simulink model "block_diagram"  (R2015b)
settings: Solver=VariableStepAuto  StartTime=0.0  StopTime=10.0  RelTol=1e-3
values from neighbouring files (symbols this model uses):
  dg = [1 1]    [script.m]
  ng = 1    [script.m]
undefined symbols (not defined in the file or in its folder): denk, numk
settings Model: Creator=EriveltonDell  LastModifiedBy=EriveltonDell

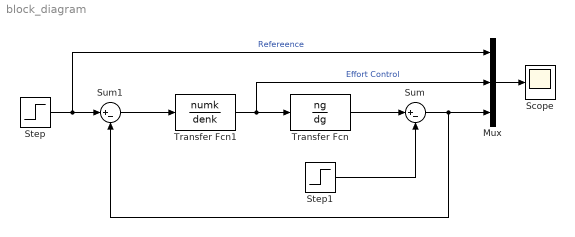
== system block_diagram ==
  Mux : Mux  Inputs=3
  Scope : Scope
  Step : Step  SampleTime=0
  Step1 : Step  Time=5  SampleTime=0
  Sum : Sum  Inputs=|+-
  Sum1 : Sum  Inputs=|+-
  Transfer Fcn : TransferFcn  Numerator=ng  Denominator=dg
  Transfer Fcn1 : TransferFcn  Numerator=numk  Denominator=denk
  wires:
  Transfer Fcn/1 -> Sum/1
  Transfer Fcn1/1 -> Mux/2, Transfer Fcn/1  "Effort Control"
  Sum1/1 -> Transfer Fcn1/1
  Step/1 -> Mux/1, Sum1/1  "Refereence"
  Mux/1 -> Scope/1
  Sum/1 -> Sum1/2, Mux/3
  Step1/1 -> Sum/2
